simulink model "airtrim"  (Simulink 3.00)
settings: Solver=ode45  StartTime=0.0  StopTime=10.0  RelTol=1e-3
libraries: airlib x1
settings Model: LoadExternalInput=on  ExternalInput=[0 1 0 0 0 0 0 0 0 0 6.7015280237240514e-017]  LoadInitialState=on  InitialState=[100;0.33384643595852526;0;0;0;0;0;0.33384643595852531;0;0;0;60]  ExtModeTrigMode=normal  ExtModeArmWhenConnect=on  LastModifiedBy=gcampa

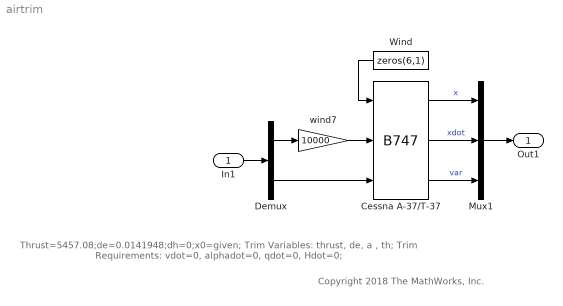
== system airtrim ==
  note: Thrust=5457.08;de=0.0141948;dh=0;x0=given;
      | Trim Variables: thrust, de, a , th;
      | Trim Requirements: vdot=0, alphadot=0, qdot=0, Hdot=0;
  note: Copyright 2018 The MathWorks, Inc.
  In1 : Inport  Port=1  PortWidth=-1  SampleTime=-1  DataType=auto
      settings: SignalType=auto
  " Cessna A-37/T-37 " : airlib/B747  GM1="[1.6673 10.3022  16.9084  10826  4509.5  15162  0 0 0   2884.9]"  CD_wind="[0.048  0.384  0  0  0]"  CL_wind="[0.2   5.15    4.1   0.5   0]"  Cm_body="[0.025   -0.7   -14.9   -1.12  0]"  CY_body="[0  -0.346  -0.0827  0.3  0.0  0.2]"  Cl_body="[0   -0.0944  -0.442  0.0926  -0.181  0.015]"  Cn_body="[0    0.1106   -0.0243   -0.139  0.0254  -0.0365]"  x0="[100  0.0130027 0   0 0 0   0 0.0130027 0   0 0 60]"
  Demux : Demux  Outputs=[6 4]
  Mux1 : Mux  Inputs=[12 12 12]
      settings: DisplayOption=none
  Wind : Constant  Orientation=left  Value=zeros(6,1)
  wind7 : Gain  Gain=10000  SaturateOnIntegerOverflow=on
  Out1 : Outport  Port=1
  wires:
  Demux/1 -> wind7/1
  In1/1 -> Demux/1
  Mux1/1 -> Out1/1
  Wind/1 -> " Cessna A-37/T-37 "/1
  wind7/1 -> " Cessna A-37/T-37 "/2
  Demux/2 -> " Cessna A-37/T-37 "/3
  " Cessna A-37/T-37 "/1 -> Mux1/1  "x"
  " Cessna A-37/T-37 "/2 -> Mux1/2  "xdot"
  " Cessna A-37/T-37 "/3 -> Mux1/3  "var"
